simulink model "harness_HFUC_8_2A"  (R2024b)
settings: Solver=ode23t  StartTime=0.0  StopTime=10.0  RelTol=1e-3
StopFcn:
  | Simulink.sdi.view;
  | Simulink.sdi.loadView('view_test_hd');
libraries: fl_lib x19, nesl_utility x8, sdl_lib x2, ssc_components x1
settings Model: Creator=upattacini  LastModifiedBy=upattacini
settings DataIOCC: SaveOutput=off  DSMLogging=off  SaveTime=off  ReturnWorkspaceOutputs=off

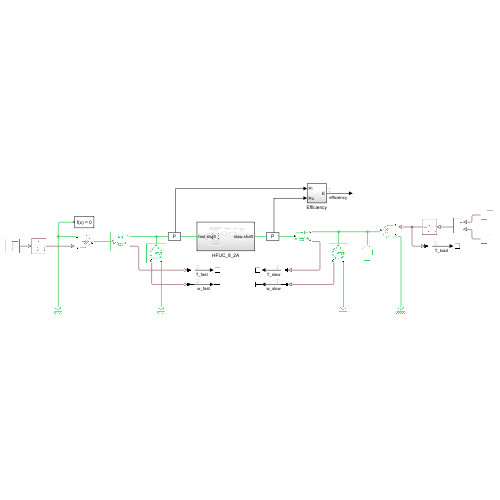
[thumbnail: Simulink's stored preview of the top-level diagram]
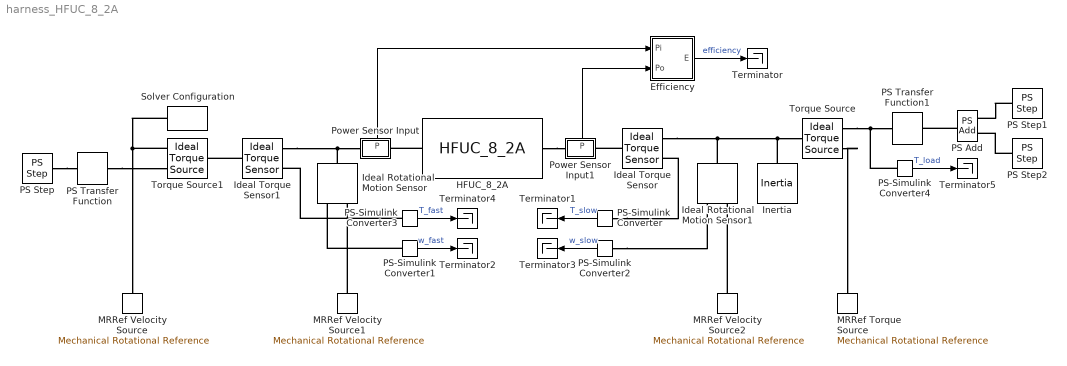
== system harness_HFUC_8_2A ==
  Efficiency : Subsystem
  HFUC_8_2A : ssc_components/Transmissions/Harmonic Drives/HFUC_8_2A  SystemSampleTime=-1  VariantActivationTime=update diagram  AllowFlexibleInterface=on  Latency=0  AutoFrameSizeCalculation=off
  Ideal Rotational Motion Sensor : fl_lib/Mechanical/Mechanical Sensors/Ideal Rotational Motion Sensor  reference=foundation.enum.MeasurementReference.difference  acceleration_port=false  velocity_port=true  position_port=false  wrap_angle=false  offset=0 rad
      settings: InternalSimscapePortConfiguration="{\"Bottom\":[],\"Left\":[{\"id\":\"R\",\"label\":\"R\",\"type\":\"foundation.mechanical.rotational.rotational\"}],\"Right\":[{\"id\":\"C\",\"label\":\"C\",\"type\":\"foundation.mechanical.rotational.rotational\"},{\"id\":\"W\",\"label\":\"W\",\"type\":\"output\"}],\"Top\":[]}"
  Ideal Rotational Motion Sensor1 : fl_lib/Mechanical/Mechanical Sensors/Ideal Rotational Motion Sensor  reference=foundation.enum.MeasurementReference.difference  acceleration_port=false  velocity_port=true  position_port=false  wrap_angle=false  offset=0 rad
      settings: InternalSimscapePortConfiguration="{\"Bottom\":[],\"Left\":[{\"id\":\"R\",\"label\":\"R\",\"type\":\"foundation.mechanical.rotational.rotational\"}],\"Right\":[{\"id\":\"C\",\"label\":\"C\",\"type\":\"foundation.mechanical.rotational.rotational\"},{\"id\":\"W\",\"label\":\"W\",\"type\":\"output\"}],\"Top\":[]}"
  Ideal Torque Sensor : fl_lib/Mechanical/Mechanical Sensors/Ideal Torque Sensor
  Ideal Torque Sensor1 : fl_lib/Mechanical/Mechanical Sensors/Ideal Torque Sensor
  Inertia : fl_lib/Mechanical/Rotational Elements/Inertia  inertia=0.2 kg*m^2  num_ports=foundation.enum.numPorts2.one  w_specify=off  w_priority=High  w=0 rad/s  w_nominal_specify=off  w_nominal_value=1  w_nominal_unit=rad/s  t_specify=off  t_priority=None  t=0 N*m  t_nominal_specify=off  t_nominal_value=1  t_nominal_unit=N*m
  MRRef Torque Source : fl_lib/Mechanical/Rotational Elements/Mechanical Rotational Reference
  MRRef Velocity Source : fl_lib/Mechanical/Rotational Elements/Mechanical Rotational Reference
  MRRef Velocity Source1 : fl_lib/Mechanical/Rotational Elements/Mechanical Rotational Reference
  MRRef Velocity Source2 : fl_lib/Mechanical/Rotational Elements/Mechanical Rotational Reference
  PS Add : fl_lib/Physical Signals/Functions/PS Add
  PS Step : fl_lib/Physical Signals/Sources/PS Step  step_time=1 s  initial_value=0 mN*m  final_value=10 mN*m
  PS Step1 : fl_lib/Physical Signals/Sources/PS Step  step_time=2 s  initial_value=0 N*m  final_value=0.1 N*m
  PS Step2 : fl_lib/Physical Signals/Sources/PS Step  step_time=4 s  initial_value=0 N*m  final_value=0.1 N*m
  PS Transfer Function : fl_lib/Physical Signals/Linear Operators/PS Transfer Function  transfer_function_type=foundation.enum.transfer_function_type.lag  T=0.25 s  T1=2 s  T2=1 s  reset_method=foundation.enum.IntegratorResetSpec.None  initial_condition_spec=foundation.enum.IntegratorICSpec.Internal  y0=0 mN*m
      settings: InternalSimscapePortConfiguration="{\"Bottom\":[],\"Left\":[{\"id\":\"U\",\"label\":\"\",\"type\":\"input\"}],\"Right\":[{\"id\":\"Y\",\"label\":\"\",\"type\":\"output\"}],\"Top\":[]}"
  PS Transfer Function1 : fl_lib/Physical Signals/Linear Operators/PS Transfer Function  transfer_function_type=foundation.enum.transfer_function_type.lag  T=0.25 s  T1=2 s  T2=1 s  reset_method=foundation.enum.IntegratorResetSpec.None  initial_condition_spec=foundation.enum.IntegratorICSpec.Internal  y0=0 N*m
      settings: InternalSimscapePortConfiguration="{\"Bottom\":[],\"Left\":[{\"id\":\"U\",\"label\":\"\",\"type\":\"input\"}],\"Right\":[{\"id\":\"Y\",\"label\":\"\",\"type\":\"output\"}],\"Top\":[]}"
  PS-Simulink Converter : nesl_utility/PS-Simulink Converter  PhysicalDomain=network_engine_domain  SubClassName=ps_output  LeftPortType=input  RightPortType=output  PseudoPeriodic=off  Frequencies=[]  VectorFormat=inherit  Unit=N*m  AffineConversion=off
  PS-Simulink Converter1 : nesl_utility/PS-Simulink Converter  PhysicalDomain=network_engine_domain  SubClassName=ps_output  LeftPortType=input  RightPortType=output  PseudoPeriodic=off  Frequencies=[]  VectorFormat=inherit  Unit=rpm  AffineConversion=off
  PS-Simulink Converter2 : nesl_utility/PS-Simulink Converter  PhysicalDomain=network_engine_domain  SubClassName=ps_output  LeftPortType=input  RightPortType=output  PseudoPeriodic=off  Frequencies=[]  VectorFormat=inherit  Unit=rpm  AffineConversion=off
  PS-Simulink Converter3 : nesl_utility/PS-Simulink Converter  PhysicalDomain=network_engine_domain  SubClassName=ps_output  LeftPortType=input  RightPortType=output  PseudoPeriodic=off  Frequencies=[]  VectorFormat=inherit  Unit=mN*m  AffineConversion=off
  PS-Simulink Converter4 : nesl_utility/PS-Simulink Converter  PhysicalDomain=network_engine_domain  SubClassName=ps_output  LeftPortType=input  RightPortType=output  PseudoPeriodic=off  Frequencies=[]  VectorFormat=inherit  Unit=N*m  AffineConversion=off
  Power Sensor Input : Subsystem
      settings: PortSchema="{\"entries\":[{\"content\":{\"sides\":[{\"content\":{\"connectorIds\":[\"LConn1\"]},\"type\":\"ConnectorPlacement.EquallySpacedRectSide\",\"uuid\":\"e0699c54-df28-4178-977a-7df40a6118cd\"},{\"content\":{\"connectorIds\":[\"RConn1\"],\"side\":\"RIGHT\"},\"type\":\"ConnectorPlacement.EquallySpacedRectSide\",\"uuid\":\"67cba640-a47c-40e4-9b66-f74b00b45e76\"},{\"content\":{\"connectorIds\":[\"Out1\"],\"side\":\"TOP\"},\"type\":\"ConnectorPlacement.EquallySpacedRectSide\",\"uuid\":\"ea664432-b525-4e00-bae7-de1e258876da\"},{\"content\":{\"side\":\"BOTTOM\"},\"type\":\"ConnectorPlacement.EquallySpacedRectSide\",\"uuid\":\"3118ccf3-5985-484f-bec3-c66d0e05ad2a\"}]},\"type\":\"ConnectorPlacement.EquallySpacedConnector\",\"uuid\":\"f48e4892-b362-478a-a103-0b200e6255c8\"}],\"packageUris\":[\"http://schema.mathworks.com/mf0/Connector/R2020b\"],\"version\":\"1.0\"}"
      mask Display: disp('P');
  Power Sensor Input1 : Subsystem
      settings: PortSchema="{\"entries\":[{\"content\":{\"sides\":[{\"content\":{\"connectorIds\":[\"LConn1\"]},\"type\":\"ConnectorPlacement.EquallySpacedRectSide\",\"uuid\":\"e0699c54-df28-4178-977a-7df40a6118cd\"},{\"content\":{\"connectorIds\":[\"RConn1\"],\"side\":\"RIGHT\"},\"type\":\"ConnectorPlacement.EquallySpacedRectSide\",\"uuid\":\"67cba640-a47c-40e4-9b66-f74b00b45e76\"},{\"content\":{\"connectorIds\":[\"Out1\"],\"side\":\"TOP\"},\"type\":\"ConnectorPlacement.EquallySpacedRectSide\",\"uuid\":\"ea664432-b525-4e00-bae7-de1e258876da\"},{\"content\":{\"side\":\"BOTTOM\"},\"type\":\"ConnectorPlacement.EquallySpacedRectSide\",\"uuid\":\"3118ccf3-5985-484f-bec3-c66d0e05ad2a\"}]},\"type\":\"ConnectorPlacement.EquallySpacedConnector\",\"uuid\":\"f48e4892-b362-478a-a103-0b200e6255c8\"}],\"packageUris\":[\"http://schema.mathworks.com/mf0/Connector/R2020b\"],\"version\":\"1.0\"}"
      mask Display: disp('P');
  Solver Configuration : nesl_utility/Solver Configuration  PhysicalDomain=network_engine_domain  SubClassName=solver  LeftPortType=input  RightPortType=generic  Tones=[]  Harmonics=[]  SimulateNoise=off  Profile=off  UseLocalSampling=off  EnableSwitchedLinearOptims=on  FrequencyDomain=off  UseCCode=off  RelTol=0.001  AbsTol=1e-06  MinStep=1e-09  ToWorkspace=off  RevertToSquareIcSolve=off  NumHomotopyIterations=100  PhasorMode=off  PhasorModeNumHarmonics=1  ConsistencySolver=NEWTON_XTOL_AFTER_FTOL  IndexReductionMethod=DerivativeReplacement  DoDC=off  ResidualTolerance=1e-9  ConsistencyTolSource=GLOBAL  ConsistencyAbsTol=0.001  ConsistencyRelTol=0.001  ConsistencyTolFactor=0.001  UseLocalSolver=off  LocalSolverChoice=NE_PARTITIONING_ADVANCER  ResolveIndetEquations=on  FunctionEvalNumThread=1  LocalSolverSampleTime=0.01  DoFixedCost=off  MaxNonlinIter=3  MaxModeIter=2  ComputeImpulses=off  ImpulseIterations=2  LinearAlgebra=auto  LinearAlgebraNumThread=0  EquationFormulation=NE_TIME_EF  DelaysMemoryBudget=1024  AutomaticFiltering=on  FilteringTimeConstant=0.001  PartitionStorageMethod=EXHAUSTIVE  PartitionMemoryBudget=1024  PartitionMethod=ROBUST  MultibodyUseLocalSolver=off  MultibodyLocalSolverChoice=ODE1  MultibodyLocalSolverSampleTime=0.001
  Terminator{,1..5} (6 alike) : Terminator
  Torque Source : fl_lib/Mechanical/Mechanical Sources/Ideal Torque Source
  Torque Source1 : fl_lib/Mechanical/Mechanical Sources/Ideal Torque Source
  wires:
  Power Sensor Input/1(P) -> Efficiency/1(Pi)
  Power Sensor Input1/1(P) -> Efficiency/2(Po)
  Efficiency/1(E) -> Terminator/1  "efficiency"
  PS-Simulink Converter/1 -> Terminator1/1  "T_slow"
  PS-Simulink Converter1/1 -> Terminator2/1  "w_fast"
  PS-Simulink Converter2/1 -> Terminator3/1  "w_slow"
  PS-Simulink Converter3/1 -> Terminator4/1  "T_fast"
  PS-Simulink Converter4/1 -> Terminator5/1  "T_load"
  connections:
  HFUC_8_2A/LConn1 -- Power Sensor Input/RConn1
  HFUC_8_2A/RConn1 -- Power Sensor Input1/LConn1
  Torque Source/RConn2 -- MRRef Torque Source/LConn1
  Ideal Torque Sensor/LConn1 -- Power Sensor Input1/RConn1
  Ideal Torque Sensor/RConn1 -- Inertia/LConn1 -- Torque Source/LConn1 -- Ideal Rotational Motion Sensor1/LConn1
  PS-Simulink Converter/LConn1 -- Ideal Torque Sensor/RConn2
  Ideal Rotational Motion Sensor/LConn1 -- Ideal Torque Sensor1/RConn1 -- Power Sensor Input/LConn1
  MRRef Velocity Source1/LConn1 -- Ideal Rotational Motion Sensor/RConn1
  PS-Simulink Converter1/LConn1 -- Ideal Rotational Motion Sensor/RConn2
  MRRef Velocity Source2/LConn1 -- Ideal Rotational Motion Sensor1/RConn1
  PS-Simulink Converter2/LConn1 -- Ideal Rotational Motion Sensor1/RConn2
  Torque Source1/RConn2 -- Solver Configuration/RConn1 -- MRRef Velocity Source/LConn1
  PS Step/RConn1 -- PS Transfer Function/LConn1
  Ideal Torque Sensor1/LConn1 -- Torque Source1/LConn1
  PS-Simulink Converter3/LConn1 -- Ideal Torque Sensor1/RConn2
  PS Transfer Function/RConn1 -- Torque Source1/RConn1
  PS-Simulink Converter4/LConn1 -- PS Transfer Function1/RConn1 -- Torque Source/RConn1
  PS Add/RConn1 -- PS Transfer Function1/LConn1
  PS Step2/RConn1 -- PS Add/LConn1
  PS Step1/RConn1 -- PS Add/LConn2

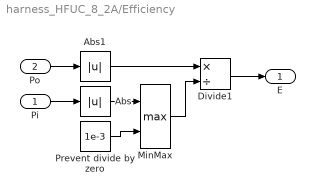
== system harness_HFUC_8_2A/Efficiency ==
  Pi : Inport
  Po : Inport  Port=2
  Abs : Abs  SaturateOnIntegerOverflow=off
  Abs1 : Abs  SaturateOnIntegerOverflow=off
  Divide1 : Product  Inputs=*/
  MinMax : MinMax  Function=max  Inputs=2
  Prevent divide by zero : Constant  Value=1e-3
  E : Outport  VectorParamsAs1DForOutWhenUnconnected=off
  wires:
  Prevent divide by zero/1 -> MinMax/2
  MinMax/1 -> Divide1/2
  Abs/1 -> MinMax/1
  Abs1/1 -> Divide1/1
  Po/1 -> Abs1/1
  Pi/1 -> Abs/1
  Divide1/1 -> E/1

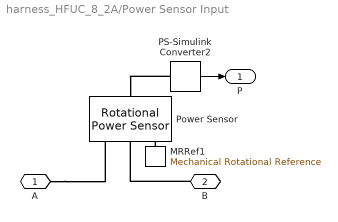
== system harness_HFUC_8_2A/Power Sensor Input ==
  MRRef1 : fl_lib/Mechanical/Rotational Elements/Mechanical Rotational Reference
  PS-Simulink Converter2 : nesl_utility/PS-Simulink Converter  PhysicalDomain=network_engine_domain  SubClassName=ps_output  LeftPortType=input  RightPortType=output  PseudoPeriodic=off  Frequencies=[]  VectorFormat=1-D array  Unit=W  AffineConversion=off
  Power Sensor : sdl_lib/Sensors/Rotational Power Sensor  measurement_type=1  averaging_period=1 s  max_frequency=1000 Hz  max_speed=1000 rpm
      settings: InternalSimscapePortConfiguration="{\"Bottom\":[],\"Left\":[{\"id\":\"S\",\"label\":\"S\",\"type\":\"foundation.mechanical.rotational.rotational\"},{\"id\":\"R\",\"label\":\"R\",\"type\":\"foundation.mechanical.rotational.rotational\"},{\"id\":\"C\",\"label\":\"C\",\"type\":\"foundation.mechanical.rotational.rotational\"}],\"Right\":[{\"id\":\"P\",\"label\":\"P\",\"type\":\"output\"}],\"Top\":[]}"
  A : PMIOPort  Side=Left
  B : PMIOPort  Port=2  Side=Right
  P : Outport
  wires:
  PS-Simulink Converter2/1 -> P/1
  connections:
  MRRef1/LConn1 -- Power Sensor/LConn3
  PS-Simulink Converter2/LConn1 -- Power Sensor/RConn1
  A/RConn1 -- Power Sensor/LConn1
  B/RConn1 -- Power Sensor/LConn2

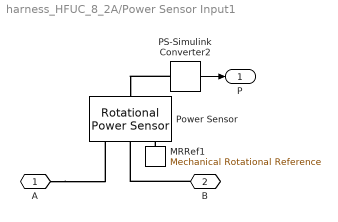
== system harness_HFUC_8_2A/Power Sensor Input1 ==
  MRRef1 : fl_lib/Mechanical/Rotational Elements/Mechanical Rotational Reference
  PS-Simulink Converter2 : nesl_utility/PS-Simulink Converter  PhysicalDomain=network_engine_domain  SubClassName=ps_output  LeftPortType=input  RightPortType=output  PseudoPeriodic=off  Frequencies=[]  VectorFormat=1-D array  Unit=W  AffineConversion=off
  Power Sensor : sdl_lib/Sensors/Rotational Power Sensor  measurement_type=1  averaging_period=1 s  max_frequency=1000 Hz  max_speed=1000 rpm
      settings: InternalSimscapePortConfiguration="{\"Bottom\":[],\"Left\":[{\"id\":\"S\",\"label\":\"S\",\"type\":\"foundation.mechanical.rotational.rotational\"},{\"id\":\"R\",\"label\":\"R\",\"type\":\"foundation.mechanical.rotational.rotational\"},{\"id\":\"C\",\"label\":\"C\",\"type\":\"foundation.mechanical.rotational.rotational\"}],\"Right\":[{\"id\":\"P\",\"label\":\"P\",\"type\":\"output\"}],\"Top\":[]}"
  A : PMIOPort  Side=Left
  B : PMIOPort  Port=2  Side=Right
  P : Outport
  wires:
  PS-Simulink Converter2/1 -> P/1
  connections:
  B/RConn1 -- Power Sensor/LConn2
  A/RConn1 -- Power Sensor/LConn1
  PS-Simulink Converter2/LConn1 -- Power Sensor/RConn1
  MRRef1/LConn1 -- Power Sensor/LConn3
